simulink model "DEC_p2015"  (R2015a)
settings: Solver=ode5  StartTime=0  StopTime=sim_time-1/sr  FixedStep=1/sr  RelTol=1e-3
values from neighbouring files (symbols this model uses):
  par = p.Results.par_fix    [balance_sim.m]
settings Model: Creator=lorenz  LastModifiedBy=lorenz
settings DataIOCC: LimitDataPoints=off  SignalLoggingSaveFormat=ModelDataLogs  SaveOutput=off  SignalLogging=off  DSMLogging=off  SaveTime=off
settings OptimizationCC: OptimizeBlockIOStorage=off  BufferReuse=off  GlobalBufferReuse=off  ExpressionFolding=off  LocalBlockOutputs=off
settings DebuggingCC: UnderspecifiedInitializationDetection=Classic  SolverPrmCheckMsg=warning  InheritedTsInSrcMsg=none  MultiTaskDSMMsg=warning  MultiTaskCondExecSysMsg=none
settings ModelReferenceCC: UpdateModelReferenceTargets=AssumeUpToDate  CheckModelReferenceTargetMessage=warning
settings RTWCC: ProfileTLC=on  RTWUseSimCustomCode=on
settings CodeAppCC: MATLABSourceComments=on

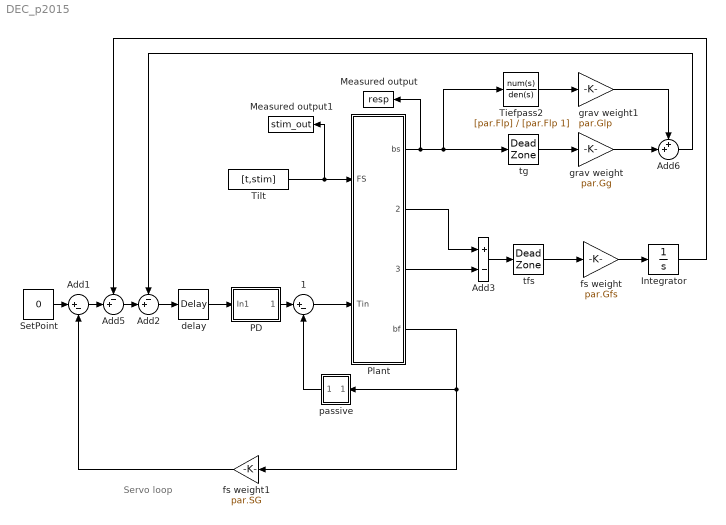
== system DEC_p2015 ==
  note: Servo loop
  " 1" : Sum  Inputs=|+-
  Add1 : Sum  Inputs=|+-
  Add2 : Sum  Inputs=-+|
  Add3 : Sum  Inputs=+-
  Add5 : Sum  Inputs=-+|
  Add6 : Sum  Inputs=++|
  Integrator : Integrator
  Measured output : ToWorkspace  VariableName=resp  SampleTime=-1
  Measured output1 : ToWorkspace  VariableName=stim_out  SampleTime=-1
  PD : Subsystem
  Plant : Subsystem
  SetPoint : Constant  Value=0
  Tiefpass2 : TransferFcn  Numerator=[par.Flp]  Denominator=[par.Flp 1]
  Tilt : FromWorkspace  VariableName=[t,stim]
  delay : TransportDelay  DelayTime=par.dt  FixedBuffer=on
  fs weight : Gain  Gain=par.Gfs
  fs weight1 : Gain  RequirementInfo={} %GIDa_9b962c78_9ae0_45e4_8b1e_11e3fb44b0b7  Gain=par.SG
  grav weight : Gain  Gain=par.Gg
  grav weight1 : Gain  Gain=par.Glp
  passive : Subsystem
  tfs : DeadZone  LowerValue=-par.tfs  UpperValue=par.tfs  LinearizeAsGain=off
  tg : DeadZone  LowerValue=-par.tg  UpperValue=par.tg  LinearizeAsGain=off
  wires:
  fs weight1/1 -> Add1/2
  PD/1(Out1) -> " 1"/1
  SetPoint/1 -> Add1/1
  tfs/1 -> fs weight/1
  fs weight/1 -> Integrator/1
  Plant/2(d bs /dt) -> Add3/1
  Plant/3(d bf / dt) -> Add3/2
  Add3/1 -> tfs/1
  Integrator/1 -> Add5/1
  grav weight/1 -> Add6/2
  Add6/1 -> Add2/1
  Tiefpass2/1 -> grav weight1/1
  grav weight1/1 -> Add6/1
  Plant/4(bf) -> fs weight1/1, passive/1(In1)
  Add2/1 -> delay/1
  Add1/1 -> Add5/2
  tg/1 -> grav weight/1
  Plant/1(bs) -> Measured output/1, Tiefpass2/1, tg/1
  " 1"/1 -> Plant/2(Tin)
  passive/1(Out1) -> " 1"/2
  Add5/1 -> Add2/2
  delay/1 -> PD/1(In1)
  Tilt/1 -> Measured output1/1, Plant/1(FS)

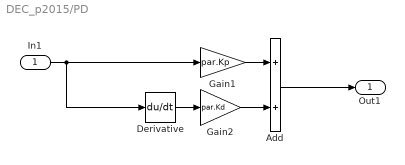
== system DEC_p2015/PD ==
  In1 : Inport
  Add : Sum
  Derivative : Derivative
  Gain1 : Gain  Gain=par.Kp
  Gain2 : Gain  Gain=par.Kd
  Out1 : Outport
  wires:
  Gain2/1 -> Add/2
  Derivative/1 -> Gain2/1
  Add/1 -> Out1/1
  In1/1 -> Derivative/1, Gain1/1
  Gain1/1 -> Add/1

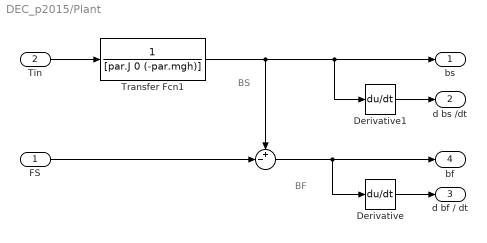
== system DEC_p2015/Plant ==
  note: BF
  note: BS
  FS : Inport
  Tin : Inport  Port=2
  " " : Sum  Inputs=+-|
  Derivative : Derivative
  Derivative1 : Derivative
  Transfer Fcn1 : TransferFcn  Denominator=[par.J 0 (-par.mgh)]
  bs : Outport
  d bs /dt : Outport  Port=2
  d bf / dt : Outport  Port=3
  bf : Outport  Port=4
  wires:
  " "/1 -> Derivative/1, bf/1
  FS/1 -> " "/2
  Tin/1 -> Transfer Fcn1/1
  Derivative1/1 -> d bs /dt/1
  Derivative/1 -> d bf / dt/1
  Transfer Fcn1/1 -> " "/1, bs/1, Derivative1/1

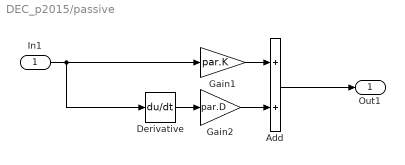
== system DEC_p2015/passive ==
  In1 : Inport
  Add : Sum
  Derivative : Derivative
  Gain1 : Gain  Gain=par.K
  Gain2 : Gain  Gain=par.D
  Out1 : Outport
  wires:
  Gain2/1 -> Add/2
  Derivative/1 -> Gain2/1
  Add/1 -> Out1/1
  In1/1 -> Derivative/1, Gain1/1
  Gain1/1 -> Add/1
